simulink model "sfcndemo_sfun_dynsize"  (Simulink 7.6)
settings: Solver=FixedStepDiscrete  StartTime=0.0  StopTime=10.0  RelTol=1e-3  AbsTol=1e-6
Description:
  | Propagated Port Dimensions C-MEX S-function
settings Model: Creator=The MathWorks Inc.  ExtModeTrigMode=oneshot  ExtModeArmWhenConnect=off  ExtModeAutoUpdateStatusClock=off
settings DataIOCC: LimitDataPoints=off
settings OptimizationCC: BlockReduction=off  BooleanDataType=off  InlineInvariantSignals=on  InitFltsAndDblsToZero=on
settings DebuggingCC: SaveWithParameterizedLinksMsg=none  SignalResolutionControl=TryResolveAllWithWarning  SolverPrmCheckMsg=none  InheritedTsInSrcMsg=none  MultiTaskDSMMsg=warning  MultiTaskCondExecSysMsg=none
settings HardwareCC: TargetUnknown=on
settings RTWCC: IncludeERTFirstTime=on
settings CodeAppCC: CustomSymbolStrFcn=$F$N$M
settings GRTTargetCC: TargetFcnLib=ansi_tfl_tmw.mat

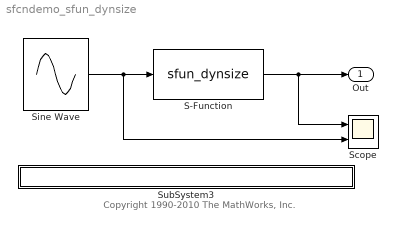
== system sfcndemo_sfun_dynsize ==
  note: Copyright 1990-2010 The MathWorks, Inc.
  S-Function : S-Function  FunctionName=sfun_dynsize  EnableBusSupport=off
      mask Type: S-function: sfun_dynsize
      mask Display:
      | plot([1 NaN 2:6 NaN 19 NaN 1 NaN 2:6 NaN 19], [NaN 0 1 1 2 2 NaN 2 NaN NaN NaN 6 5 5 4 4 NaN 4  NaN]);
      | disp('Dynamic sized vector');
  Scope : Scope  NumInputPorts=2
      settings: TimeRange=10  YMin=-10~-4  YMax=10~4
  Sine Wave : Sin  Amplitude=1:4  SampleTime=0
  SubSystem3 : Subsystem  mask{filename=sfun_dynsize.c}
      mask init:
      | x=sfundemo_maskdisp;
      settings: AttributesFormatString=\n  OpenFcn=sfundemo_openfcn
      mask Display: disp(x);
  Out : Outport  InitialOutput=0
  wires:
  S-Function/1 -> Out/1, Scope/1
  Sine Wave/1 -> S-Function/1, Scope/2

== system sfcndemo_sfun_dynsize/SubSystem3 ==
